simulink model "Last"  (R2024b)
settings: Solver=VariableStepAuto  StartTime=0.0  StopTime=10.0  RelTol=1e-3
values from neighbouring files (symbols this model uses):
  b = 0.00002    (= 2e-05)    [Lab2.m]    (also in Last.m = 0.5; lab2_2.m = 25; untitled.m)
  J = 4*10^-6    (= 4e-06)    [Lab2.m]    (also in Last.m = 2; untitled.m)
  Kb = 0.04    [Lab2.m]    (also in Last.m = 0.1; untitled.m)
  Kt = 0.04    [Lab2.m]    (also in Last.m = 10; untitled.m)
  Ra = 1    [Last.m]    (also in untitled.m = 8)
settings Model: Creator=Abdullah  LastModifiedBy=Abdullah

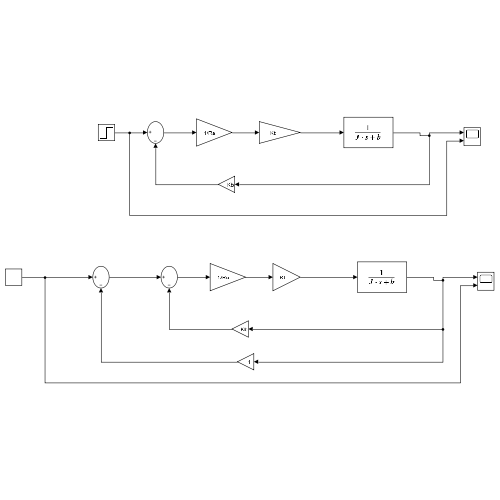
[thumbnail: Simulink's stored preview of the top-level diagram]
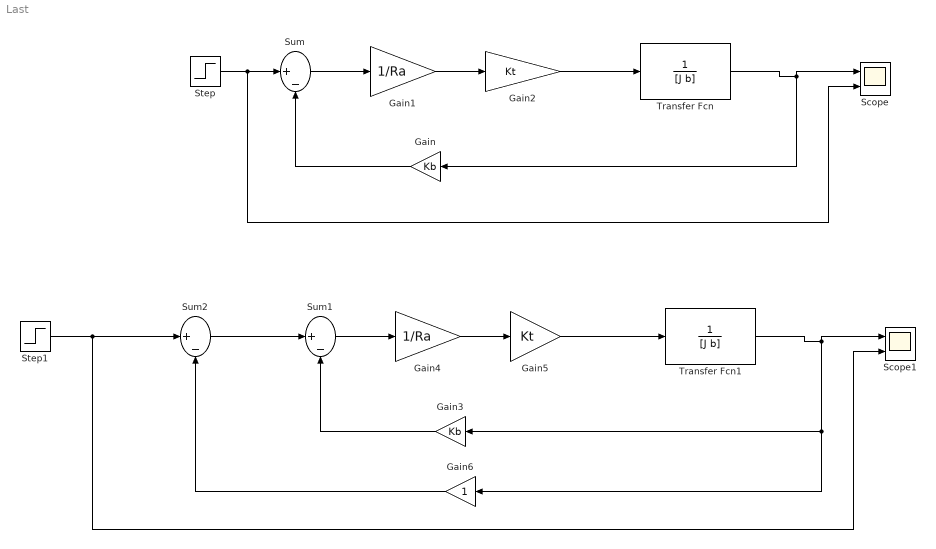
== system Last ==
  Gain : Gain  Gain=Kb
  Gain1 : Gain  Gain=1/Ra
  Gain2 : Gain  Gain=Kt
  Gain3 : Gain  Gain=Kb
  Gain4 : Gain  Gain=1/Ra
  Gain5 : Gain  Gain=Kt
  Gain6 : Gain
  Scope : Scope  NumInputPorts=2
  Scope1 : Scope  NumInputPorts=2
  Step : Step  SampleTime=0
  Step1 : Step  SampleTime=0
  Sum : Sum  Inputs=|+-
  Sum1 : Sum  Inputs=|+-
  Sum2 : Sum  Inputs=|+-
  Transfer Fcn : TransferFcn  Denominator=[J b]
  Transfer Fcn1 : TransferFcn  Denominator=[J b]
  wires:
  Transfer Fcn/1 -> Gain/1, Scope/1
  Sum/1 -> Gain1/1
  Gain1/1 -> Gain2/1
  Gain2/1 -> Transfer Fcn/1
  Step/1 -> Scope/2, Sum/1
  Gain/1 -> Sum/2
  Gain4/1 -> Gain5/1
  Gain5/1 -> Transfer Fcn1/1
  Gain3/1 -> Sum1/2
  Transfer Fcn1/1 -> Gain6/1, Gain3/1, Scope1/1
  Sum1/1 -> Gain4/1
  Sum2/1 -> Sum1/1
  Step1/1 -> Scope1/2, Sum2/1
  Gain6/1 -> Sum2/2
